simulink model "model_one"  (R2026a)
settings: Solver=VariableStepAuto  StopTime=20
values from neighbouring files (symbols this model uses):
  b = 30    [Model 1 MATLAB file.m]    (also in Model 2 MATLAB file.m = 300)
  c = 100    [Model 1 MATLAB file.m]    (also in Model 2 MATLAB file.m = 10000)
  m = 300    [Model 1 MATLAB file.m]    (also in Model 2 MATLAB file.m)
settings Model: Creator=Muhammad Zaid  LastModifiedBy=Muhammad Zaid

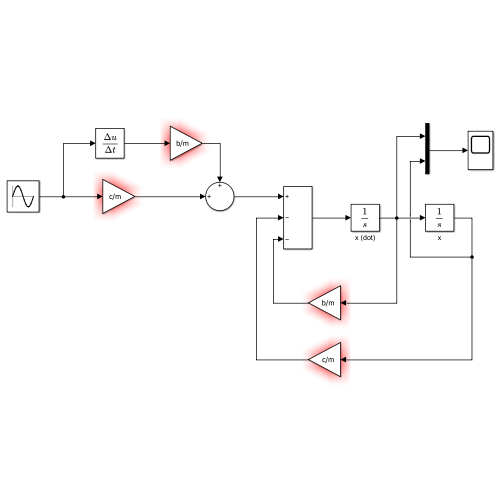
[thumbnail: Simulink's stored preview of the top-level diagram]
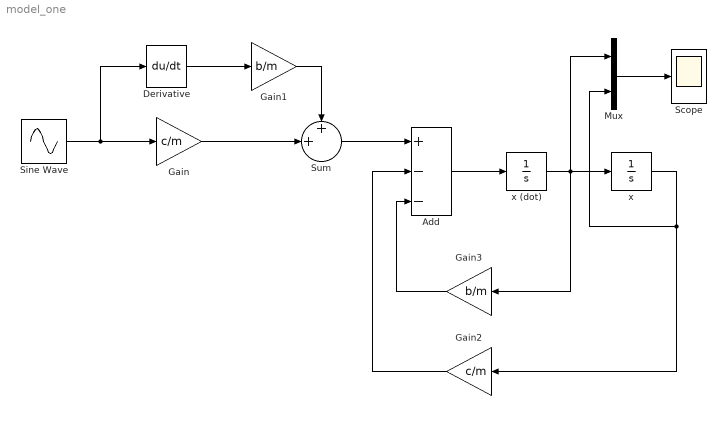
== system model_one ==
  Add : Sum  Inputs=+--
  Derivative : Derivative
  Gain : Gain  Gain=c/m
  Gain1 : Gain  Gain=b/m
  Gain2 : Gain  Gain=c/m
  Gain3 : Gain  Gain=b/m
  Mux : Mux  Inputs=2
  Scope : Scope
      settings: ActiveDisplayYMinimum=-1.3243260312771046  ActiveDisplayYMaximum=1.3210649773148777
  Sine Wave : Sin  SampleTime=0
  Sum : Sum  Inputs=++|
  x : Integrator  InitialCondition=0.2
  x (dot) : Integrator  InitialCondition=-0.3
  wires:
  Gain/1 -> Sum/2
  x (dot)/1 -> Mux/1, x/1, Gain3/1
  Mux/1 -> Scope/1
  Sine Wave/1 -> Derivative/1, Gain/1
  Gain2/1 -> Add/2
  Gain1/1 -> Sum/1
  Gain3/1 -> Add/3
  x/1 -> Mux/2, Gain2/1
  Sum/1 -> Add/1
  Add/1 -> x (dot)/1
  Derivative/1 -> Gain1/1
